simulink model "ODE1_zad2"  (Simulink 6.3)
settings: Solver=ode45  StartTime=0.0  StopTime=0.5  RelTol=1e-3
settings Model: LastModifiedBy=Ms1

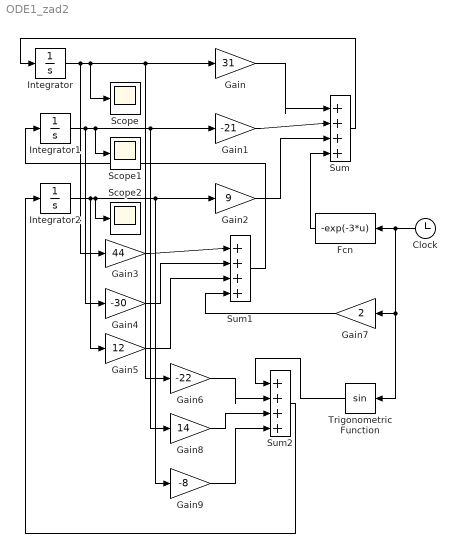
== system ODE1_zad2 ==
  Clock : Clock
      settings: Decimation=10
  Fcn : Fcn  Orientation=left  Expr=-exp(-3*u)
  Gain : Gain  Gain=31  SaturateOnIntegerOverflow=on
  Gain1 : Gain  Gain=-21  SaturateOnIntegerOverflow=on
  Gain2 : Gain  Gain=9  SaturateOnIntegerOverflow=on
  Gain3 : Gain  Gain=44  SaturateOnIntegerOverflow=on
  Gain4 : Gain  Gain=-30  SaturateOnIntegerOverflow=on
  Gain5 : Gain  Gain=12  SaturateOnIntegerOverflow=on
  Gain6 : Gain  Gain=-22  SaturateOnIntegerOverflow=on
  Gain7 : Gain  Orientation=left  Gain=2  SaturateOnIntegerOverflow=on
  Gain8 : Gain  Gain=14  SaturateOnIntegerOverflow=on
  Gain9 : Gain  Gain=-8  SaturateOnIntegerOverflow=on
  Integrator : Integrator  InitialCondition=-2
  Integrator1 : Integrator  InitialCondition=1
  Integrator2 : Integrator
  Scope : Scope
  Scope1 : Scope
  Scope2 : Scope
      settings: SaveName=ScopeData2
  Sum : Sum  Inputs=|++++  SaturateOnIntegerOverflow=on  InputSameDT=on
  Sum1 : Sum  Inputs=|++++  SaturateOnIntegerOverflow=on  InputSameDT=on
  Sum2 : Sum  Inputs=|++++  SaturateOnIntegerOverflow=on  InputSameDT=on
  Trigonometric Function : Trigonometry  Orientation=left
  wires:
  Integrator/1 -> Gain3/1, Gain/1, Gain6/1, Scope/1
  Integrator1/1 -> Gain4/1, Gain1/1, Gain8/1, Scope1/1
  Integrator2/1 -> Gain5/1, Gain2/1, Gain9/1, Scope2/1
  Gain/1 -> Sum/1
  Gain1/1 -> Sum/2
  Gain2/1 -> Sum/3
  Fcn/1 -> Sum/4
  Sum/1 -> Integrator/1
  Clock/1 -> Fcn/1, Gain7/1, Trigonometric Function/1
  Gain3/1 -> Sum1/1
  Gain4/1 -> Sum1/2
  Gain5/1 -> Sum1/3
  Gain7/1 -> Sum1/4
  Sum1/1 -> Integrator1/1
  Sum2/1 -> Integrator2/1
  Gain9/1 -> Sum2/4
  Gain8/1 -> Sum2/3
  Gain6/1 -> Sum2/2
  Trigonometric Function/1 -> Sum2/1
